simulink model "Truck_trailer_Observer_based"  (Simulink 9.3)
settings: Solver=ode45  StartTime=0.0  StopTime=60  RelTol=1e-10  EnableMultiTasking=on
values from neighbouring files (symbols this model uses):
  a = 0.7    [forsimution.m]
  A1 = [-a*v*tba/(L*t0), 0, 0;a*v*tba/(L*t0), 0, 0;a*v*v*tba*tba/(2*L*t0), v*tba/t0, 0]    [forsimution.m]
  A2 = [-a*v*tba/(L*t0), 0, 0;a*v*tba/(L*t0), 0, 0;a*c*v*v*tba*tba/(2*L*t0), c*v*tba/t0, 0]    [forsimution.m]
  A_tao_1 = [-(1-a)*v*tba/(L*t0), 0, 0;(1-a)*v*tba/(L*t0), 0, 0;(1-a)*v*v*tba*tba/(2*L*t0), 0, 0;]    [forsimution.m]
  A_tao_2 = [-(1-a)*v*tba/(L*t0), 0, 0;(1-a)*v*tba/(L*t0), 0, 0;(1-a)*c*v*v*tba*tba/(2*L*t0), 0, 0;]    [forsimution.m]
  B1 = [v*tba/(l*t0);0;0]    [forsimution.m]
  B2 = B1    [forsimution.m]
  Bw1 = [0.1;0.1;0.1]    [forsimution.m]
  Bw2 = [0.1;0.1;0.1]    [forsimution.m]
  C1 = [4.9 -2 0.04]    [forsimution.m]
  C2 = [4.9 -2 0.04]    [forsimution.m]
  E1 = [0.1 0 0]    [forsimution.m]
  E2 = [0.1 0 0]    [forsimution.m]
  E_tao_1 = [0.1 0 0]    [forsimution.m]
  K1 = [2.3490   -1.0090    0.0456]    [forsimution.m]
  K2 = [1.2632   -0.2942    0.0222]    [forsimution.m]
  L = 5.5    [forsimution.m]
  L1 = [0.3658;-2.4454;0.6900]    [forsimution.m]
  L2 = [0.6258;0.5985;2.1471]    [forsimution.m]
  tba = 2.0    (= 2)    [forsimution.m]
  v = -1.0    (= -1)    [forsimution.m]
  x0 = [-0.5*pi;0.1*pi;0.5]    [forsimution.m]
  x01 = [-0.5*pi;0.1*pi;0.5]    [forsimution.m]
libraries: commnoisgen2 x2
settings Model: Creator=user  LastModifiedBy=Shamrooz
settings OptimizationCC: ExpressionDepthLimit=2147483647  InitFltsAndDblsToZero=on
settings DebuggingCC: SaveWithParameterizedLinksMsg=none  SolverPrmCheckMsg=warning  StateNameClashWarn=warning
settings GRTTargetCC: TargetFcnLib=ansi_tfl_tmw.mat  GeneratePreprocessorConditionals=Disable all

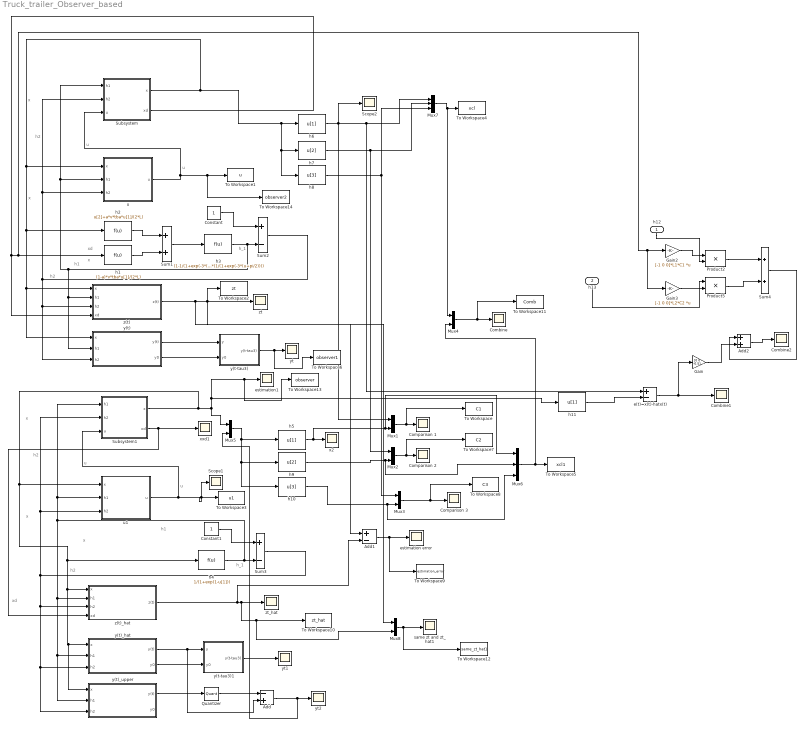
== system Truck_trailer_Observer_based ==
  note: h_1
  note: x
  note: xd
  note: h2
  note: h1
  note: h2
  note: x
  note: x
  note: u
  note: u
  note: h_1
  note: x
  note: xd
  note: h2
  note: h1
  note: h2
  note: x
  note: x
  note: u
  note: u
  h12 : Inport
  h13 : Inport  Port=2
  Add : Sum  Inputs=-+
  Add1 : Sum  Inputs=+-
  Add2 : Sum
  Combine : Scope
  Combine1 : Scope
  Combine2 : Scope
  "Comparison 1 " : Scope
  Comparison 2 : Scope
  Comparison 3 : Scope
  Constant : Constant
  Constant1 : Constant
  Gain : Gain  Gain=[0 0 -0.5]
  Gain2 : Gain  Gain=[-1 0 0]*L1*C1  Multiplication=Matrix(K*u)
  Gain3 : Gain  Gain=[-1 0 0]*L2*C2  Multiplication=Matrix(K*u)
  Mux{1..5,8} (6 alike) : Mux  Inputs=2
  Mux6 : Mux  Inputs=3
  Mux7 : Mux  Inputs=3
  Product2 : Product  SaturateOnIntegerOverflow=on  OutDataTypeStr=Inherit: Same as first input
  Product5 : Product  SaturateOnIntegerOverflow=on  OutDataTypeStr=Inherit: Same as first input
  Quantizer : Quantizer  QuantizationInterval=0.001  SampleTime=0.08
  Scope1 : Scope
  Scope2 : Scope
  Subsystem : Subsystem
  Subsystem1 : Subsystem
  Sum1 : Sum
  Sum2 : Sum  Inputs=+-
  Sum3 : Sum  Inputs=+-
  Sum4 : Sum
  To Workspace : ToWorkspace  VariableName=C1  SampleTime=-1
  To Workspace1 : ToWorkspace  VariableName=u  SampleTime=-1
  To Workspace10 : ToWorkspace  VariableName=zt_hat  SampleTime=-1
  To Workspace11 : ToWorkspace  VariableName=Comb  SampleTime=-1
  To Workspace12 : ToWorkspace  VariableName=same_zt_hat1  SampleTime=-1
  To Workspace13 : ToWorkspace  VariableName=observer  SampleTime=-1
  To Workspace14 : ToWorkspace  VariableName=observer2  SampleTime=-1
  To Workspace2 : ToWorkspace  VariableName=zt  SampleTime=-1
  To Workspace3 : ToWorkspace  VariableName=u1  SampleTime=-1
  To Workspace4 : ToWorkspace  VariableName=xcl  SampleTime=-1
  To Workspace5 : ToWorkspace  VariableName=xcl1  SampleTime=-1
  To Workspace6 : ToWorkspace  VariableName=observer1  SampleTime=-1
  To Workspace7 : ToWorkspace  VariableName=C2  SampleTime=-1
  To Workspace8 : ToWorkspace  VariableName=C3  SampleTime=-1
  To Workspace9 : ToWorkspace  VariableName=estimation_error  SampleTime=-1
  e(t)=x(t)-hatx(t) : Sum  Inputs=+-
  estimation error : Scope
  estimation1 : Scope
  h1 : Fcn  Expr=(1-a)*v*tba*u[1]/(2*L)
  h10 : Fcn  Expr=u[3]
  h11 : Fcn  Expr=u[1]
  h2 : Fcn  Expr=u[2]+a*v*tba*u[1]/(2*L)
  h3 : Fcn  Expr=(1-1/(1+exp(-3*(u-pi/2))))*(1/(1+exp(-3*(u+pi/2))))
  h4 : Fcn  Expr=1/(1+exp(1-u[1]))
  h5 : Fcn  Expr=u[1]
  h6 : Fcn  Expr=u[1]
  h7 : Fcn  Expr=u[2]
  h8 : Fcn  Expr=u[3]
  h9 : Fcn  Expr=u[2]
  same zt and zt_hat1 : Scope
  u : Subsystem
  u1 : Subsystem
  x2 : Scope
  xxd1 : Scope
  y(t) : Subsystem
  y(t)_hat : Subsystem
  y(t)_upper : Subsystem
  y(t-tau3) : Subsystem
  y(t-tau3)1 : Subsystem
  yt : Scope
  yt1 : Scope
  yt2 : Scope
  z(t) : Subsystem
  z(t)_hat : Subsystem
  zt : Scope
  zt_hat : Scope
  wires:
  Subsystem/1(x) -> h8/1, h7/1, h6/1, u/1(x), y(t)/1(x), z(t)/1(x), h2/1
  u/1(u) -> Subsystem/3(u), To Workspace14/1, To Workspace1/1
  h2/1 -> Sum1/1
  h1/1 -> Sum1/2
  Sum1/1 -> h3/1
  h3/1 -> Sum2/2, y(t)/2(h1), z(t)/2(h1), Subsystem/1(h1), u/2(h1)
  Constant/1 -> Sum2/1
  Subsystem/2(xd) -> z(t)/4(xd), Gain3/1, Gain2/1, h1/1
  Sum2/1 -> y(t)/3(h2), z(t)/3(h2), Subsystem/2(h2), u/3(h2)
  z(t)/1(z(t)) -> Mux8/1, Add1/1, To Workspace2/1, zt/1
  y(t)/1(y(t)) -> y(t-tau3)/1("y ")
  y(t)/2(y0) -> y(t-tau3)/2(y0)
  y(t-tau3)/1(y(t-tau3)) -> To Workspace6/1, yt/1
  Constant1/1 -> Sum3/1
  Sum3/1 -> Subsystem1/2(h2), u1/3(h2), y(t)_upper/3(h2), y(t)_hat/3(h2), z(t)_hat/3(h2)
  h4/1 -> Sum3/2, Subsystem1/1(h1), u1/2(h1), y(t)_upper/2(h1), y(t)_hat/2(h1), z(t)_hat/2(h1)
  Subsystem1/2(xd) -> z(t)_hat/4(xd), xxd1/1
  z(t)_hat/1(z(t)) -> Add1/2, Mux8/2, To Workspace10/1, zt_hat/1
  y(t)_hat/2(y0) -> y(t-tau3)1/2(y0)
  y(t)_hat/1(y(t)) -> Add/2, y(t-tau3)1/1("y ")
  y(t-tau3)1/1(y(t-tau3)) -> yt1/1
  u1/1(u) -> To Workspace3/1, Scope1/1, Subsystem1/3(u)
  Subsystem1/1(x) -> Mux5/1, h11/1, To Workspace13/1, estimation1/1, u1/1(x), h4/1, y(t)_upper/1(x), y(t)_hat/1(x), z(t)_hat/1(x)
  h5/1 -> Mux6/1, Mux1/2, x2/1
  Add1/1 -> To Workspace9/1, estimation error/1
  Mux1/1 -> To Workspace/1, "Comparison 1 "/1
  Mux2/1 -> To Workspace7/1, Comparison 2/1
  h9/1 -> Mux6/2, Mux2/2
  h7/1 -> Mux7/2, Mux2/1
  h8/1 -> Mux7/3, Mux3/1
  Add/1 -> Mux5/2, yt2/1
  Mux4/1 -> To Workspace11/1, Combine/1
  y(t)_upper/1(y(t)) -> Quantizer/1
  Quantizer/1 -> Add/1
  Mux5/1 -> h10/1, h9/1, h5/1
  Mux3/1 -> To Workspace8/1, Comparison 3/1
  h10/1 -> Mux6/3, Mux3/2
  Mux7/1 -> Mux4/1, To Workspace4/1
  Mux6/1 -> Mux4/2, To Workspace5/1
  Mux8/1 -> To Workspace12/1, same zt and zt_hat1/1
  h6/1 -> e(t)=x(t)-hatx(t)/1, Mux7/1, Scope2/1, Mux1/1
  h11/1 -> e(t)=x(t)-hatx(t)/2
  Add2/1 -> Combine2/1
  h13/1 -> Product5/2
  e(t)=x(t)-hatx(t)/1 -> Gain/1, Combine1/1
  h12/1 -> Product2/2
  Gain2/1 -> Product2/1
  Product2/1 -> Sum4/1
  Gain3/1 -> Product5/1
  Product5/1 -> Sum4/2
  Gain/1 -> Add2/2
  Sum4/1 -> Add2/1

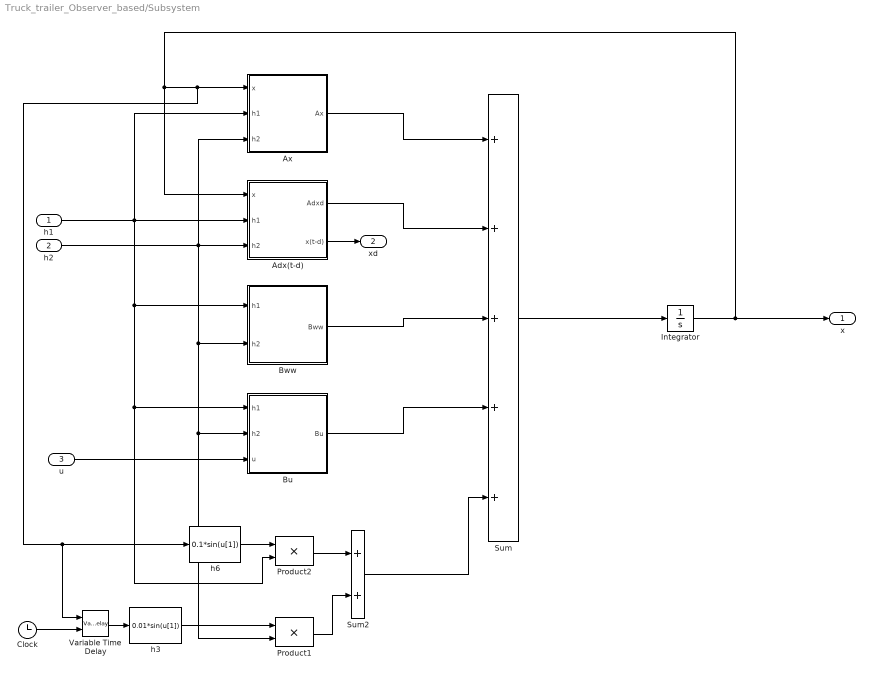
== system Truck_trailer_Observer_based/Subsystem ==
  h1 : Inport
  h2 : Inport  Port=2
  u : Inport  Port=3
  Adx(t-d) : Subsystem
  Ax : Subsystem
  Bu : Subsystem
  Bww : Subsystem
  Clock : Clock
  Integrator : Integrator  InitialCondition=x0
  Product1 : Product  SaturateOnIntegerOverflow=on  OutDataTypeStr=Inherit: Same as first input
  Product2 : Product  SaturateOnIntegerOverflow=on  OutDataTypeStr=Inherit: Same as first input
  Sum : Sum  Inputs=+++++
  Sum2 : Sum
  Variable Time Delay : VariableTransportDelay  MaximumDelay=10
  h3 : Fcn  Expr=0.01*sin(u[1])
  h6 : Fcn  Expr=0.1*sin(u[1])
  x : Outport
  xd : Outport  Port=2
  wires:
  Ax/1(Ax) -> Sum/1
  Adx(t-d)/1(Adxd) -> Sum/2
  Bww/1(Bww) -> Sum/3
  Bu/1(Bu) -> Sum/4
  Adx(t-d)/2(x(t-d)) -> xd/1
  Sum/1 -> Integrator/1
  Integrator/1 -> x/1, Variable Time Delay/1, h6/1, Ax/1(x), Adx(t-d)/1(x)
  u/1 -> Bu/3(u)
  h1/1 -> Ax/2(h1), Adx(t-d)/2(h1), Bww/1(h1), Product2/2, Bu/1(h1)
  h2/1 -> Adx(t-d)/3(h2), Ax/3(h2), Bww/2(h2), Bu/2(h2), Product1/2
  h6/1 -> Product2/1
  Product2/1 -> Sum2/1
  Sum2/1 -> Sum/5
  Product1/1 -> Sum2/2
  h3/1 -> Product1/1
  Variable Time Delay/1 -> h3/1
  Clock/1 -> Variable Time Delay/2

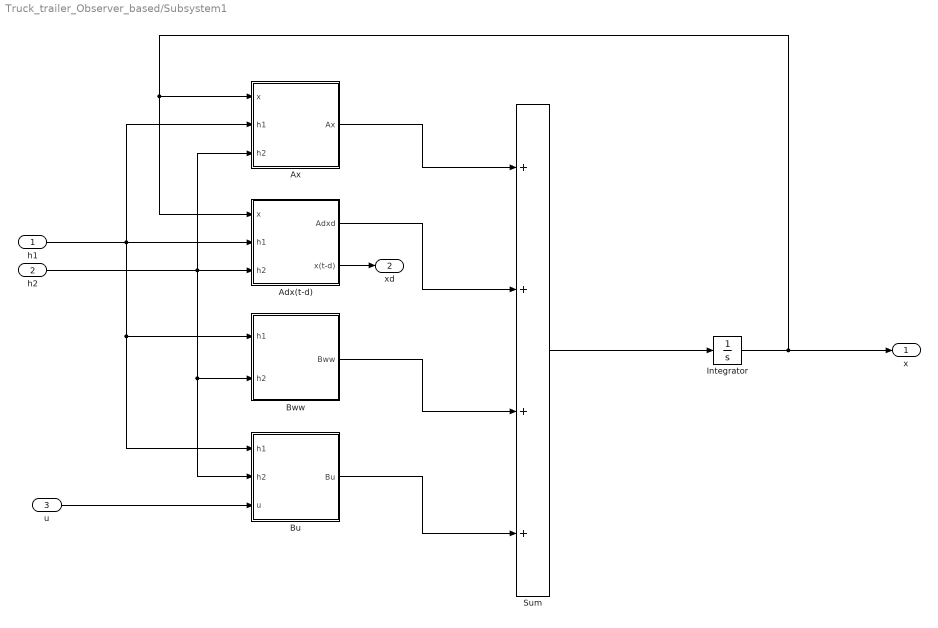
== system Truck_trailer_Observer_based/Subsystem1 ==
  h1 : Inport
  h2 : Inport  Port=2
  u : Inport  Port=3
  Adx(t-d) : Subsystem
  Ax : Subsystem
  Bu : Subsystem
  Bww : Subsystem
  Integrator : Integrator  InitialCondition=x0
  Sum : Sum  Inputs=++++
  x : Outport
  xd : Outport  Port=2
  wires:
  Ax/1(Ax) -> Sum/1
  Adx(t-d)/1(Adxd) -> Sum/2
  Bww/1(Bww) -> Sum/3
  Bu/1(Bu) -> Sum/4
  Adx(t-d)/2(x(t-d)) -> xd/1
  Sum/1 -> Integrator/1
  Integrator/1 -> x/1, Ax/1(x), Adx(t-d)/1(x)
  u/1 -> Bu/3(u)
  h1/1 -> Ax/2(h1), Adx(t-d)/2(h1), Bww/1(h1), Bu/1(h1)
  h2/1 -> Adx(t-d)/3(h2), Ax/3(h2), Bww/2(h2), Bu/2(h2)

== system Truck_trailer_Observer_based/u ==
  note: x
  x : Inport
  h1 : Inport  Port=2
  h2 : Inport  Port=3
  Gain1 : Gain  Gain=K1  Multiplication=Matrix(K*u)
  Gain3 : Gain  Gain=K2  Multiplication=Matrix(K*u)
  Product2 : Product  SaturateOnIntegerOverflow=on  OutDataTypeStr=Inherit: Same as first input
  Product5 : Product  SaturateOnIntegerOverflow=on  OutDataTypeStr=Inherit: Same as first input
  Sum2 : Sum
  u : Outport
  wires:
  Gain1/1 -> Product2/1
  x/1 -> Gain1/1, Gain3/1
  Sum2/1 -> u/1
  Product2/1 -> Sum2/1
  Product5/1 -> Sum2/2
  Gain3/1 -> Product5/1
  h1/1 -> Product2/2
  h2/1 -> Product5/2

== system Truck_trailer_Observer_based/u1 ==
  note: x
  x : Inport
  h1 : Inport  Port=2
  h2 : Inport  Port=3
  Gain1 : Gain  Gain=K1  Multiplication=Matrix(K*u)
  Gain3 : Gain  Gain=K2  Multiplication=Matrix(K*u)
  Product2 : Product  SaturateOnIntegerOverflow=on  OutDataTypeStr=Inherit: Same as first input
  Product5 : Product  SaturateOnIntegerOverflow=on  OutDataTypeStr=Inherit: Same as first input
  Sum2 : Sum
  u : Outport
  wires:
  Gain1/1 -> Product2/1
  x/1 -> Gain1/1, Gain3/1
  Sum2/1 -> u/1
  Product2/1 -> Sum2/1
  Product5/1 -> Sum2/2
  Gain3/1 -> Product5/1
  h1/1 -> Product2/2
  h2/1 -> Product5/2

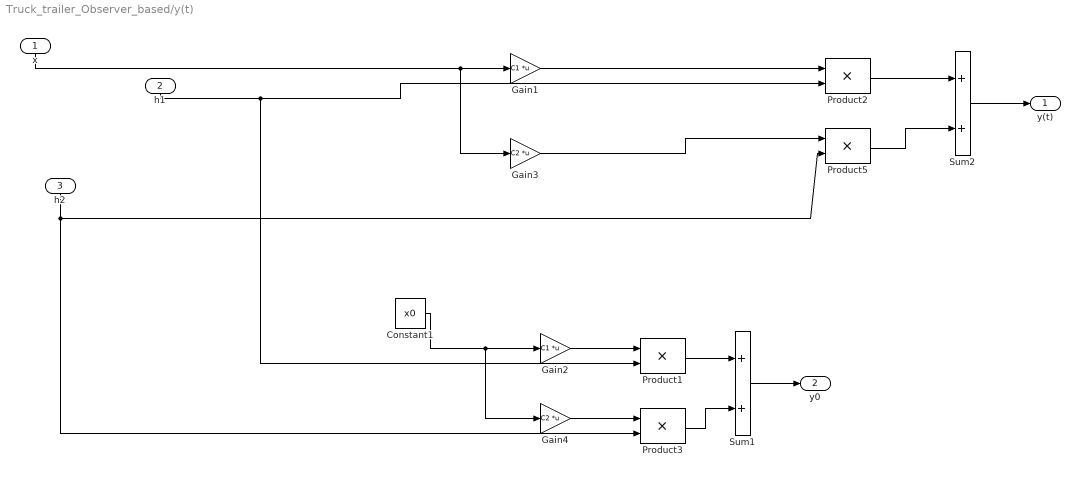
== system Truck_trailer_Observer_based/y(t) ==
  x : Inport
  h1 : Inport  Port=2
  h2 : Inport  Port=3
  Constant1 : Constant  Value=x0
  Gain1 : Gain  Gain=C1  Multiplication=Matrix(K*u)
  Gain2 : Gain  Gain=C1  Multiplication=Matrix(K*u)
  Gain3 : Gain  Gain=C2  Multiplication=Matrix(K*u)
  Gain4 : Gain  Gain=C2  Multiplication=Matrix(K*u)
  Product{1..3,5} (4 alike) : Product  SaturateOnIntegerOverflow=on  OutDataTypeStr=Inherit: Same as first input
  Sum1 : Sum
  Sum2 : Sum
  y(t) : Outport
  y0 : Outport  Port=2
  wires:
  h2/1 -> Product5/2, Product3/2
  x/1 -> Gain1/1, Gain3/1
  h1/1 -> Product2/2, Product1/2
  Gain1/1 -> Product2/1
  Sum2/1 -> y(t)/1
  Product2/1 -> Sum2/1
  Product5/1 -> Sum2/2
  Gain3/1 -> Product5/1
  Constant1/1 -> Gain2/1, Gain4/1
  Gain2/1 -> Product1/1
  Gain4/1 -> Product3/1
  Product1/1 -> Sum1/1
  Product3/1 -> Sum1/2
  Sum1/1 -> y0/1

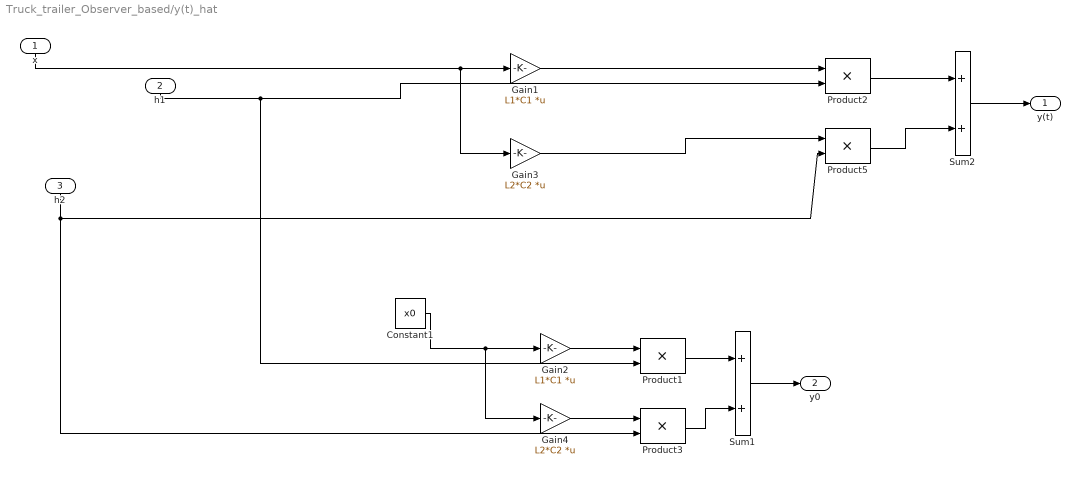
== system Truck_trailer_Observer_based/y(t)_hat ==
  x : Inport
  h1 : Inport  Port=2
  h2 : Inport  Port=3
  Constant1 : Constant  Value=x0
  Gain1 : Gain  Gain=L1*C1  Multiplication=Matrix(K*u)
  Gain2 : Gain  Gain=L1*C1  Multiplication=Matrix(K*u)
  Gain3 : Gain  Gain=L2*C2  Multiplication=Matrix(K*u)
  Gain4 : Gain  Gain=L2*C2  Multiplication=Matrix(K*u)
  Product{1..3,5} (4 alike) : Product  SaturateOnIntegerOverflow=on  OutDataTypeStr=Inherit: Same as first input
  Sum1 : Sum
  Sum2 : Sum
  y(t) : Outport
  y0 : Outport  Port=2
  wires:
  h2/1 -> Product5/2, Product3/2
  x/1 -> Gain1/1, Gain3/1
  h1/1 -> Product2/2, Product1/2
  Gain1/1 -> Product2/1
  Sum2/1 -> y(t)/1
  Product2/1 -> Sum2/1
  Product5/1 -> Sum2/2
  Gain3/1 -> Product5/1
  Constant1/1 -> Gain2/1, Gain4/1
  Gain2/1 -> Product1/1
  Gain4/1 -> Product3/1
  Product1/1 -> Sum1/1
  Product3/1 -> Sum1/2
  Sum1/1 -> y0/1

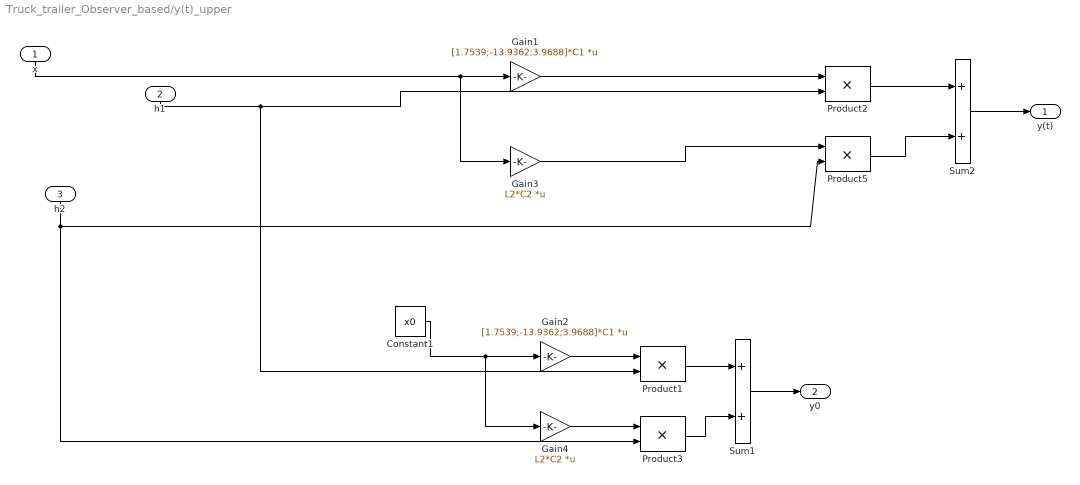
== system Truck_trailer_Observer_based/y(t)_upper ==
  x : Inport
  h1 : Inport  Port=2
  h2 : Inport  Port=3
  Constant1 : Constant  Value=x0
  Gain1 : Gain  Gain=[1.7539;-13.9362;3.9688]*C1  Multiplication=Matrix(K*u)
  Gain2 : Gain  Gain=[1.7539;-13.9362;3.9688]*C1  Multiplication=Matrix(K*u)
  Gain3 : Gain  Gain=L2*C2  Multiplication=Matrix(K*u)
  Gain4 : Gain  Gain=L2*C2  Multiplication=Matrix(K*u)
  Product{1..3,5} (4 alike) : Product  SaturateOnIntegerOverflow=on  OutDataTypeStr=Inherit: Same as first input
  Sum1 : Sum
  Sum2 : Sum
  y(t) : Outport
  y0 : Outport  Port=2
  wires:
  h2/1 -> Product5/2, Product3/2
  x/1 -> Gain1/1, Gain3/1
  h1/1 -> Product2/2, Product1/2
  Gain1/1 -> Product2/1
  Sum2/1 -> y(t)/1
  Product2/1 -> Sum2/1
  Product5/1 -> Sum2/2
  Gain3/1 -> Product5/1
  Constant1/1 -> Gain2/1, Gain4/1
  Gain2/1 -> Product1/1
  Gain4/1 -> Product3/1
  Product1/1 -> Sum1/1
  Product3/1 -> Sum1/2
  Sum1/1 -> y0/1

== system Truck_trailer_Observer_based/y(t-tau3) ==
  note: tau3
  "y " : Inport
  y0 : Inport  Port=2
  Clock : Clock
  Sum4 : Sum  Inputs=+-
  Switch : Switch  Criteria=u2 > Threshold  SaturateOnIntegerOverflow=on
  Variable Time Delay : VariableTransportDelay  MaximumDelay=tao_3
  h4 : Fcn  Expr=2+2*sin(0.25*u)
  xft : Scope
  y(t-tau3) : Outport
  wires:
  "y "/1 -> Variable Time Delay/1
  Sum4/1 -> Switch/2
  Variable Time Delay/1 -> Switch/1
  y0/1 -> Switch/3
  h4/1 -> Variable Time Delay/2, Sum4/2, xft/1
  Switch/1 -> y(t-tau3)/1
  Clock/1 -> h4/1, Sum4/1

== system Truck_trailer_Observer_based/y(t-tau3)1 ==
  note: tau3
  "y " : Inport
  y0 : Inport  Port=2
  Clock : Clock
  Sum4 : Sum  Inputs=+-
  Switch : Switch  Criteria=u2 > Threshold  SaturateOnIntegerOverflow=on
  Variable Time Delay : VariableTransportDelay  MaximumDelay=tao_3
  h4 : Fcn  Expr=2+2*sin(0.25*u)
  xft : Scope
  y(t-tau3) : Outport
  wires:
  "y "/1 -> Variable Time Delay/1
  Sum4/1 -> Switch/2
  Variable Time Delay/1 -> Switch/1
  y0/1 -> Switch/3
  h4/1 -> Variable Time Delay/2, Sum4/2, xft/1
  Switch/1 -> y(t-tau3)/1
  Clock/1 -> h4/1, Sum4/1

== system Truck_trailer_Observer_based/z(t) ==
  note: z
  x : Inport
  h1 : Inport  Port=2
  h2 : Inport  Port=3
  xd : Inport  Port=4
  Edfx(t-d) : Subsystem
  Ex : Subsystem
  Sum3 : Sum
  z(t) : Outport
  wires:
  h1/1 -> Ex/2(h1), Edfx(t-d)/2(h1)
  xd/1 -> Edfx(t-d)/1(xd)
  x/1 -> Ex/1(x)
  h2/1 -> Ex/3(h2), Edfx(t-d)/3(h2)
  Edfx(t-d)/1(Edxd) -> Sum3/2
  Ex/1(Ex) -> Sum3/1
  Sum3/1 -> z(t)/1

== system Truck_trailer_Observer_based/z(t)_hat ==
  note: z
  x : Inport
  h1 : Inport  Port=2
  h2 : Inport  Port=3
  xd : Inport  Port=4
  Edfx(t-d) : Subsystem
  Ex : Subsystem
  Sum3 : Sum
  z(t) : Outport
  wires:
  h1/1 -> Ex/2(h1), Edfx(t-d)/2(h1)
  xd/1 -> Edfx(t-d)/1(xd)
  x/1 -> Ex/1(x)
  h2/1 -> Ex/3(h2), Edfx(t-d)/3(h2)
  Edfx(t-d)/1(Edxd) -> Sum3/2
  Ex/1(Ex) -> Sum3/1
  Sum3/1 -> z(t)/1

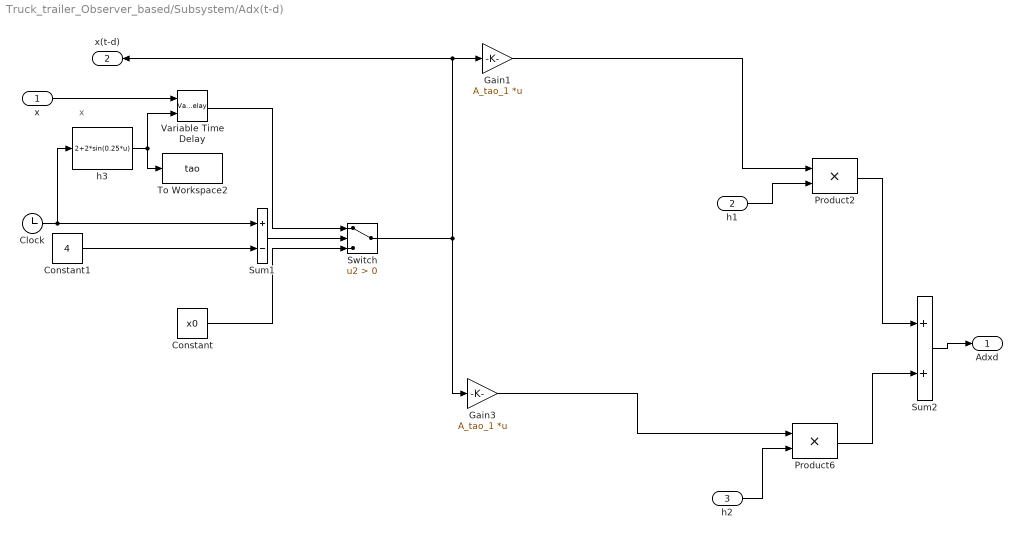
== system Truck_trailer_Observer_based/Subsystem/Adx(t-d) ==
  note: x
  x : Inport
  h1 : Inport  Port=2
  h2 : Inport  Port=3
  Clock : Clock
  Constant : Constant  Value=x0
  Constant1 : Constant  Value=4
  Gain1 : Gain  Gain=A_tao_1  Multiplication=Matrix(K*u)
  Gain3 : Gain  Gain=A_tao_1  Multiplication=Matrix(K*u)
  Product2 : Product  SaturateOnIntegerOverflow=on  OutDataTypeStr=Inherit: Same as first input
  Product6 : Product  SaturateOnIntegerOverflow=on  OutDataTypeStr=Inherit: Same as first input
  Sum1 : Sum  Inputs=+-
  Sum2 : Sum
  Switch : Switch  Criteria=u2 > Threshold  SaturateOnIntegerOverflow=on
  To Workspace2 : ToWorkspace  VariableName=tao  SampleTime=-1
  Variable Time Delay : VariableTransportDelay  MaximumDelay=10
  h3 : Fcn  Expr=2+2*sin(0.25*u)
  Adxd : Outport
  x(t-d) : Outport  Port=2
  wires:
  x/1 -> Variable Time Delay/1
  Gain1/1 -> Product2/1
  Product2/1 -> Sum2/1
  Product6/1 -> Sum2/2
  Sum2/1 -> Adxd/1
  Gain3/1 -> Product6/1
  h1/1 -> Product2/2
  h2/1 -> Product6/2
  Clock/1 -> Sum1/1, h3/1
  Constant1/1 -> Sum1/2
  Sum1/1 -> Switch/2
  Variable Time Delay/1 -> Switch/1
  Constant/1 -> Switch/3
  Switch/1 -> Gain3/1, x(t-d)/1, Gain1/1
  h3/1 -> Variable Time Delay/2, To Workspace2/1

== system Truck_trailer_Observer_based/Subsystem/Ax ==
  note: x
  x : Inport
  h1 : Inport  Port=2
  h2 : Inport  Port=3
  Gain1 : Gain  Gain=A1  Multiplication=Matrix(K*u)
  Gain3 : Gain  Gain=A2  Multiplication=Matrix(K*u)
  Product2 : Product  SaturateOnIntegerOverflow=on  OutDataTypeStr=Inherit: Same as first input
  Product5 : Product  SaturateOnIntegerOverflow=on  OutDataTypeStr=Inherit: Same as first input
  Sum2 : Sum
  Ax : Outport
  wires:
  Gain1/1 -> Product2/1
  x/1 -> Gain1/1, Gain3/1
  Sum2/1 -> Ax/1
  Product2/1 -> Sum2/1
  Product5/1 -> Sum2/2
  Gain3/1 -> Product5/1
  h1/1 -> Product2/2
  h2/1 -> Product5/2

== system Truck_trailer_Observer_based/Subsystem/Bu ==
  h1 : Inport
  h2 : Inport  Port=2
  u : Inport  Port=3
  Gain1 : Gain  Gain=B1
  Gain3 : Gain  Gain=B2
  Product2 : Product  SaturateOnIntegerOverflow=on  OutDataTypeStr=Inherit: Same as first input
  Product5 : Product  SaturateOnIntegerOverflow=on  OutDataTypeStr=Inherit: Same as first input
  Sum2 : Sum
  Bu : Outport
  wires:
  Gain1/1 -> Product2/1
  Sum2/1 -> Bu/1
  Product2/1 -> Sum2/1
  Product5/1 -> Sum2/2
  Gain3/1 -> Product5/1
  h1/1 -> Product2/2
  h2/1 -> Product5/2
  u/1 -> Gain1/1, Gain3/1

== system Truck_trailer_Observer_based/Subsystem/Bww ==
  note: w
  h1 : Inport
  h2 : Inport  Port=2
  Clock : Clock
  Gain1 : Gain  Gain=Bw1
  Gain3 : Gain  Gain=Bw2
  Noise Generator : Subsystem
  Product2 : Product  SaturateOnIntegerOverflow=on  OutDataTypeStr=Inherit: Same as first input
  Product5 : Product  SaturateOnIntegerOverflow=on  OutDataTypeStr=Inherit: Same as first input
  Sum2 : Sum
  Uniform Noise Generator1 : commnoisgen2/Uniform Noise Generator  low=-0.05  up=0.05  seed=31  Ts=0.01  frameBased=off  sampPerFrame=1  orient=off  outDataType=double
      settings: SourceProductName=Communications Toolbox  SourceProductBaseCode=CM
  Bww : Outport
  wires:
  h2/1 -> Product5/2
  h1/1 -> Product2/2
  Gain3/1 -> Product5/1
  Product5/1 -> Sum2/2
  Product2/1 -> Sum2/1
  Sum2/1 -> Bww/1
  Gain1/1 -> Product2/1
  Uniform Noise Generator1/1 -> Gain3/1, Gain1/1

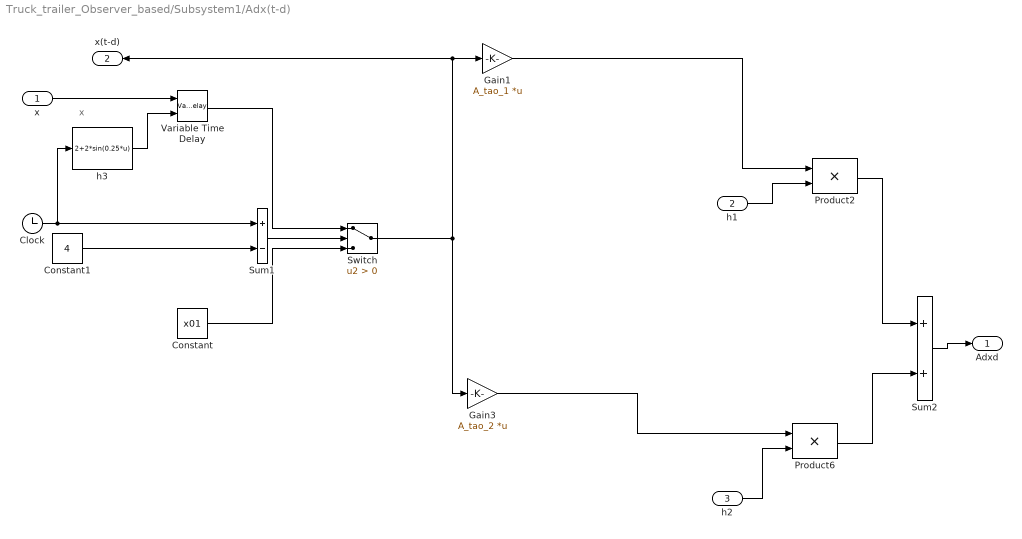
== system Truck_trailer_Observer_based/Subsystem1/Adx(t-d) ==
  note: x
  x : Inport
  h1 : Inport  Port=2
  h2 : Inport  Port=3
  Clock : Clock
  Constant : Constant  Value=x01
  Constant1 : Constant  Value=4
  Gain1 : Gain  Gain=A_tao_1  Multiplication=Matrix(K*u)
  Gain3 : Gain  Gain=A_tao_2  Multiplication=Matrix(K*u)
  Product2 : Product  SaturateOnIntegerOverflow=on  OutDataTypeStr=Inherit: Same as first input
  Product6 : Product  SaturateOnIntegerOverflow=on  OutDataTypeStr=Inherit: Same as first input
  Sum1 : Sum  Inputs=+-
  Sum2 : Sum
  Switch : Switch  Criteria=u2 > Threshold  SaturateOnIntegerOverflow=on
  Variable Time Delay : VariableTransportDelay  MaximumDelay=10
  h3 : Fcn  Expr=2+2*sin(0.25*u)
  Adxd : Outport
  x(t-d) : Outport  Port=2
  wires:
  x/1 -> Variable Time Delay/1
  Gain1/1 -> Product2/1
  Product2/1 -> Sum2/1
  Product6/1 -> Sum2/2
  Sum2/1 -> Adxd/1
  Gain3/1 -> Product6/1
  h1/1 -> Product2/2
  h2/1 -> Product6/2
  Clock/1 -> Sum1/1, h3/1
  Constant1/1 -> Sum1/2
  Sum1/1 -> Switch/2
  Variable Time Delay/1 -> Switch/1
  Constant/1 -> Switch/3
  Switch/1 -> Gain3/1, x(t-d)/1, Gain1/1
  h3/1 -> Variable Time Delay/2

== system Truck_trailer_Observer_based/Subsystem1/Ax ==
  note: x
  x : Inport
  h1 : Inport  Port=2
  h2 : Inport  Port=3
  Gain1 : Gain  Gain=A1  Multiplication=Matrix(K*u)
  Gain3 : Gain  Gain=A2  Multiplication=Matrix(K*u)
  Product2 : Product  SaturateOnIntegerOverflow=on  OutDataTypeStr=Inherit: Same as first input
  Product5 : Product  SaturateOnIntegerOverflow=on  OutDataTypeStr=Inherit: Same as first input
  Sum2 : Sum
  Ax : Outport
  wires:
  Gain1/1 -> Product2/1
  x/1 -> Gain1/1, Gain3/1
  Sum2/1 -> Ax/1
  Product2/1 -> Sum2/1
  Product5/1 -> Sum2/2
  Gain3/1 -> Product5/1
  h1/1 -> Product2/2
  h2/1 -> Product5/2

== system Truck_trailer_Observer_based/Subsystem1/Bu ==
  h1 : Inport
  h2 : Inport  Port=2
  u : Inport  Port=3
  Gain1 : Gain  Gain=B1
  Gain3 : Gain  Gain=B2
  Product2 : Product  SaturateOnIntegerOverflow=on  OutDataTypeStr=Inherit: Same as first input
  Product5 : Product  SaturateOnIntegerOverflow=on  OutDataTypeStr=Inherit: Same as first input
  Sum2 : Sum
  Bu : Outport
  wires:
  Gain1/1 -> Product2/1
  Sum2/1 -> Bu/1
  Product2/1 -> Sum2/1
  Product5/1 -> Sum2/2
  Gain3/1 -> Product5/1
  h1/1 -> Product2/2
  h2/1 -> Product5/2
  u/1 -> Gain1/1, Gain3/1

== system Truck_trailer_Observer_based/Subsystem1/Bww ==
  note: w
  h1 : Inport
  h2 : Inport  Port=2
  Gain1 : Gain  Gain=Bw1
  Gain3 : Gain  Gain=Bw2
  Noise Generator : Subsystem
  Product2 : Product  SaturateOnIntegerOverflow=on  OutDataTypeStr=Inherit: Same as first input
  Product5 : Product  SaturateOnIntegerOverflow=on  OutDataTypeStr=Inherit: Same as first input
  Sum2 : Sum
  Uniform Noise Generator1 : commnoisgen2/Uniform Noise Generator  low=-0.05  up=0.05  seed=31  Ts=0.01  frameBased=off  sampPerFrame=1  orient=off  outDataType=double
      settings: SourceProductName=Communications Toolbox  SourceProductBaseCode=CM
  Bww : Outport
  wires:
  h2/1 -> Product5/2
  h1/1 -> Product2/2
  Gain3/1 -> Product5/1
  Product5/1 -> Sum2/2
  Product2/1 -> Sum2/1
  Sum2/1 -> Bww/1
  Gain1/1 -> Product2/1
  Uniform Noise Generator1/1 -> Gain1/1, Gain3/1

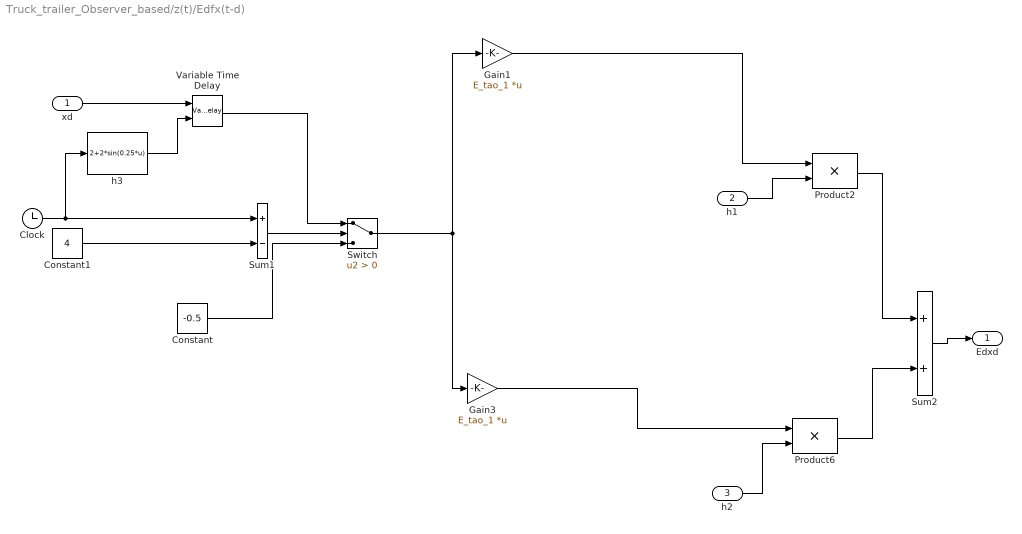
== system Truck_trailer_Observer_based/z(t)/Edfx(t-d) ==
  xd : Inport
  h1 : Inport  Port=2
  h2 : Inport  Port=3
  Clock : Clock
  Constant : Constant  Value=-0.5
  Constant1 : Constant  Value=4
  Gain1 : Gain  Gain=E_tao_1  Multiplication=Matrix(K*u)
  Gain3 : Gain  Gain=E_tao_1  Multiplication=Matrix(K*u)
  Product2 : Product  SaturateOnIntegerOverflow=on  OutDataTypeStr=Inherit: Same as first input
  Product6 : Product  SaturateOnIntegerOverflow=on  OutDataTypeStr=Inherit: Same as first input
  Sum1 : Sum  Inputs=+-
  Sum2 : Sum
  Switch : Switch  Criteria=u2 > Threshold  SaturateOnIntegerOverflow=on
  Variable Time Delay : VariableTransportDelay  MaximumDelay=0.7
  h3 : Fcn  Expr=2+2*sin(0.25*u)
  Edxd : Outport
  wires:
  Switch/1 -> Gain3/1, Gain1/1
  Constant/1 -> Switch/3
  Sum1/1 -> Switch/2
  Constant1/1 -> Sum1/2
  Clock/1 -> h3/1, Sum1/1
  h2/1 -> Product6/2
  h1/1 -> Product2/2
  Gain3/1 -> Product6/1
  Sum2/1 -> Edxd/1
  Product6/1 -> Sum2/2
  Product2/1 -> Sum2/1
  Gain1/1 -> Product2/1
  h3/1 -> Variable Time Delay/2
  Variable Time Delay/1 -> Switch/1
  xd/1 -> Variable Time Delay/1

== system Truck_trailer_Observer_based/z(t)/Ex ==
  note: x
  x : Inport
  h1 : Inport  Port=2
  h2 : Inport  Port=3
  Gain1 : Gain  Gain=E1  Multiplication=Matrix(K*u)
  Gain3 : Gain  Gain=E2  Multiplication=Matrix(K*u)
  Product2 : Product  SaturateOnIntegerOverflow=on  OutDataTypeStr=Inherit: Same as first input
  Product5 : Product  SaturateOnIntegerOverflow=on  OutDataTypeStr=Inherit: Same as first input
  Sum2 : Sum
  Ex : Outport
  wires:
  h2/1 -> Product5/2
  h1/1 -> Product2/2
  Gain3/1 -> Product5/1
  Product5/1 -> Sum2/2
  Product2/1 -> Sum2/1
  Sum2/1 -> Ex/1
  x/1 -> Gain3/1, Gain1/1
  Gain1/1 -> Product2/1

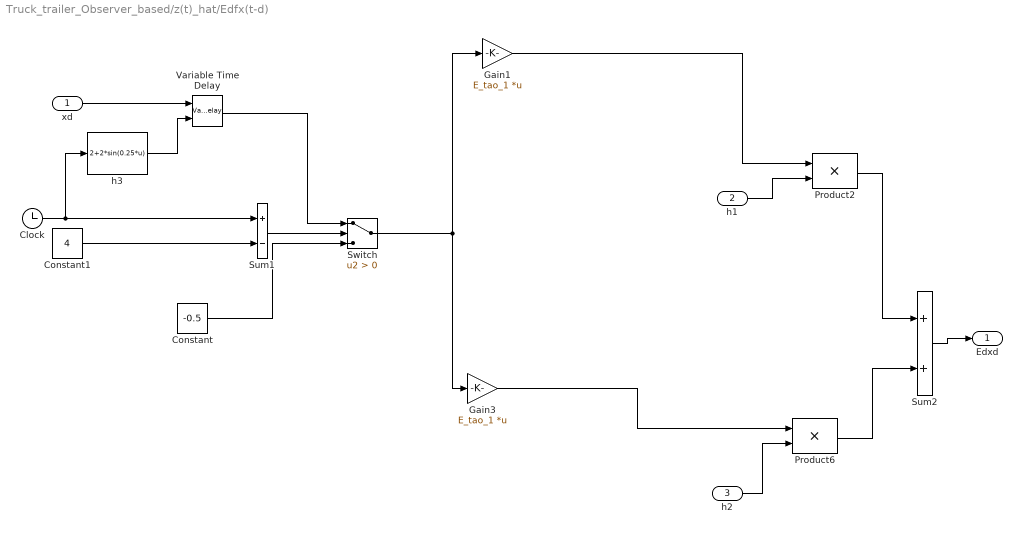
== system Truck_trailer_Observer_based/z(t)_hat/Edfx(t-d) ==
  xd : Inport
  h1 : Inport  Port=2
  h2 : Inport  Port=3
  Clock : Clock
  Constant : Constant  Value=-0.5
  Constant1 : Constant  Value=4
  Gain1 : Gain  Gain=E_tao_1  Multiplication=Matrix(K*u)
  Gain3 : Gain  Gain=E_tao_1  Multiplication=Matrix(K*u)
  Product2 : Product  SaturateOnIntegerOverflow=on  OutDataTypeStr=Inherit: Same as first input
  Product6 : Product  SaturateOnIntegerOverflow=on  OutDataTypeStr=Inherit: Same as first input
  Sum1 : Sum  Inputs=+-
  Sum2 : Sum
  Switch : Switch  Criteria=u2 > Threshold  SaturateOnIntegerOverflow=on
  Variable Time Delay : VariableTransportDelay  MaximumDelay=0.7
  h3 : Fcn  Expr=2+2*sin(0.25*u)
  Edxd : Outport
  wires:
  Switch/1 -> Gain3/1, Gain1/1
  Constant/1 -> Switch/3
  Sum1/1 -> Switch/2
  Constant1/1 -> Sum1/2
  Clock/1 -> h3/1, Sum1/1
  h2/1 -> Product6/2
  h1/1 -> Product2/2
  Gain3/1 -> Product6/1
  Sum2/1 -> Edxd/1
  Product6/1 -> Sum2/2
  Product2/1 -> Sum2/1
  Gain1/1 -> Product2/1
  h3/1 -> Variable Time Delay/2
  Variable Time Delay/1 -> Switch/1
  xd/1 -> Variable Time Delay/1

== system Truck_trailer_Observer_based/z(t)_hat/Ex ==
  note: x
  x : Inport
  h1 : Inport  Port=2
  h2 : Inport  Port=3
  Gain1 : Gain  Gain=E1  Multiplication=Matrix(K*u)
  Gain3 : Gain  Gain=E2  Multiplication=Matrix(K*u)
  Product2 : Product  SaturateOnIntegerOverflow=on  OutDataTypeStr=Inherit: Same as first input
  Product5 : Product  SaturateOnIntegerOverflow=on  OutDataTypeStr=Inherit: Same as first input
  Sum2 : Sum
  Ex : Outport
  wires:
  h2/1 -> Product5/2
  h1/1 -> Product2/2
  Gain3/1 -> Product5/1
  Product5/1 -> Sum2/2
  Product2/1 -> Sum2/1
  Sum2/1 -> Ex/1
  x/1 -> Gain3/1, Gain1/1
  Gain1/1 -> Product2/1

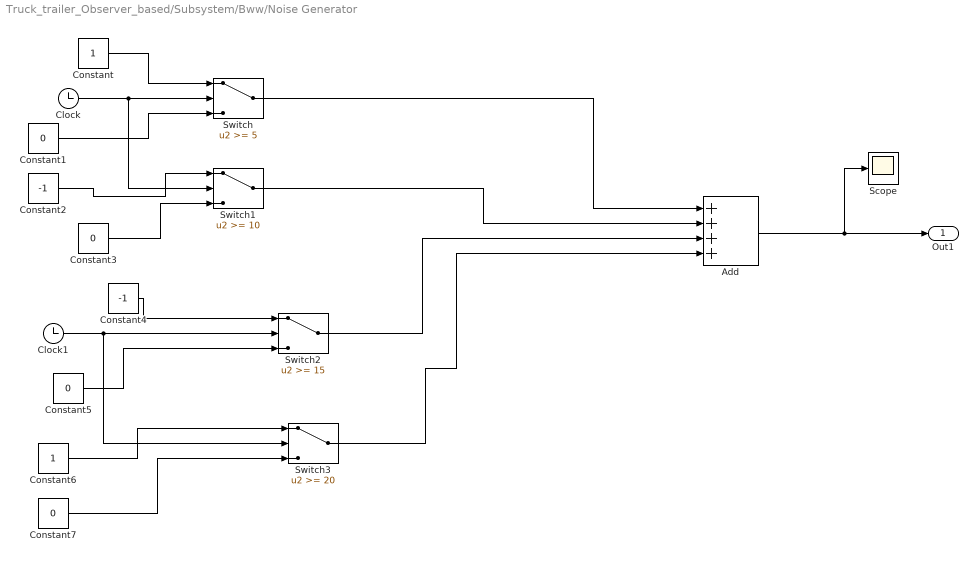
== system Truck_trailer_Observer_based/Subsystem/Bww/Noise Generator ==
  Add : Sum  Inputs=++++
  Clock : Clock
  Clock1 : Clock
  Constant : Constant
  Constant{1,3,5,7} (4 alike) : Constant  Value=0
  Constant2 : Constant  Value=-1
  Constant4 : Constant  Value=-1
  Constant6 : Constant
  Scope : Scope
  Switch : Switch  Threshold=5
  Switch1 : Switch  Threshold=10
  Switch2 : Switch  Threshold=15
  Switch3 : Switch  Threshold=20
  Out1 : Outport
  wires:
  Constant6/1 -> Switch3/1
  Switch3/1 -> Add/4
  Constant3/1 -> Switch1/3
  Switch/1 -> Add/1
  Constant5/1 -> Switch2/3
  Constant4/1 -> Switch2/1
  Clock1/1 -> Switch3/2, Switch2/2
  Constant7/1 -> Switch3/3
  Switch2/1 -> Add/3
  Switch1/1 -> Add/2
  Constant/1 -> Switch/1
  Add/1 -> Scope/1, Out1/1
  Constant1/1 -> Switch/3
  Clock/1 -> Switch1/2, Switch/2
  Constant2/1 -> Switch1/1

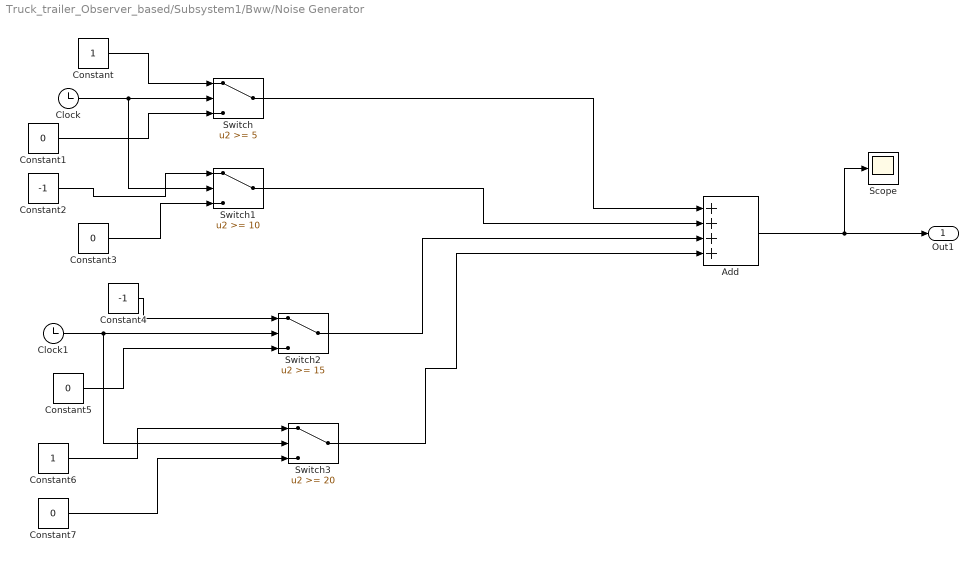
== system Truck_trailer_Observer_based/Subsystem1/Bww/Noise Generator ==
  Add : Sum  Inputs=++++
  Clock : Clock
  Clock1 : Clock
  Constant : Constant
  Constant{1,3,5,7} (4 alike) : Constant  Value=0
  Constant2 : Constant  Value=-1
  Constant4 : Constant  Value=-1
  Constant6 : Constant
  Scope : Scope
  Switch : Switch  Threshold=5
  Switch1 : Switch  Threshold=10
  Switch2 : Switch  Threshold=15
  Switch3 : Switch  Threshold=20
  Out1 : Outport
  wires:
  Constant6/1 -> Switch3/1
  Switch3/1 -> Add/4
  Constant3/1 -> Switch1/3
  Switch/1 -> Add/1
  Constant5/1 -> Switch2/3
  Constant4/1 -> Switch2/1
  Clock1/1 -> Switch3/2, Switch2/2
  Constant7/1 -> Switch3/3
  Switch2/1 -> Add/3
  Switch1/1 -> Add/2
  Constant/1 -> Switch/1
  Add/1 -> Scope/1, Out1/1
  Constant1/1 -> Switch/3
  Clock/1 -> Switch1/2, Switch/2
  Constant2/1 -> Switch1/1
